simulink model "thorp"  (R2016b)
settings: Solver=VariableStepAuto  StartTime=0.0  StopTime=10.0  RelTol=1e-3
libraries: simulink x1
settings Model: Creator=charAn  LastModifiedBy=charAn

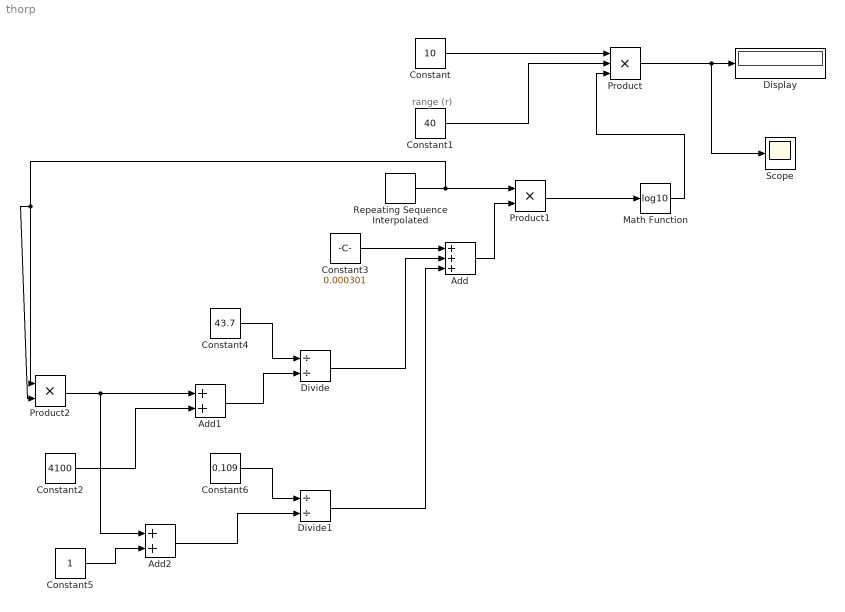
== system thorp ==
  note: range (r)
  Add : Sum  Inputs=+++
  Add1 : Sum
  Add2 : Sum
  Constant : Constant  Value=10
  Constant1 : Constant  Value=40
  Constant2 : Constant  Value=4100
  Constant3 : Constant  Value=0.000301
  Constant4 : Constant  Value=43.7
  Constant5 : Constant
  Constant6 : Constant  Value=0.109
  Display : Display
  Divide : Product  Inputs=//
  Divide1 : Product  Inputs=//
  Math Function : Math  Operator=log10  SaturateOnIntegerOverflow=on
  Product : Product  Inputs=3
  Product1 : Product
  Product2 : Product
  Repeating Sequence Interpolated : simulink/Sources/Repeating Sequence Interpolated  OutValues=[0 1000 2000 3000 4000 5000 6000 7000 8000 9000 10000]  TimeValues=[0 10 20 30 40 50 60 70 80 90 100]  LookUpMeth=Interpolation-Use End Values  tsamp=0.01  OutMin=[]  OutMax=[]  OutDataTypeStr=double  OutputDataTypeScalingMode=double  OutDataType=fixdt(0,8)  OutScaling=2^-10
  Scope : Scope
  wires:
  Constant/1 -> Product/1
  Constant1/1 -> Product/2
  Math Function/1 -> Product/3
  Product/1 -> Scope/1, Display/1
  Add/1 -> Product1/2
  Product1/1 -> Math Function/1
  Constant3/1 -> Add/1
  Constant4/1 -> Divide/1
  Divide/1 -> Add/2
  Constant6/1 -> Divide1/1
  Divide1/1 -> Add/3
  Repeating Sequence Interpolated/1 -> Product2/2, Product2/1, Product1/1
  Product2/1 -> Add2/1, Add1/1
  Constant2/1 -> Add1/2
  Add1/1 -> Divide/2
  Constant5/1 -> Add2/2
  Add2/1 -> Divide1/2
